simulink subsystem "Day4_5_Scenario_1"  (R2024a)
settings: Solver=VariableStepAuto  StartTime=0.0  StopTime=10.0  RelTol=1e-3
libraries: CarMaker4SL x12, slpidlib x1
settings Model: Creator=junhyung.cha  LastModifiedBy=User

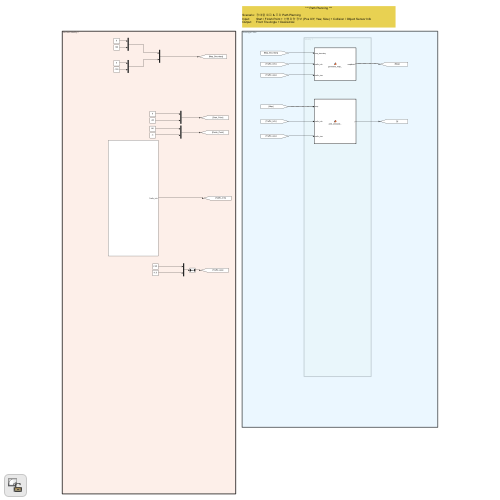
[thumbnail: Simulink's stored preview of the top-level diagram]
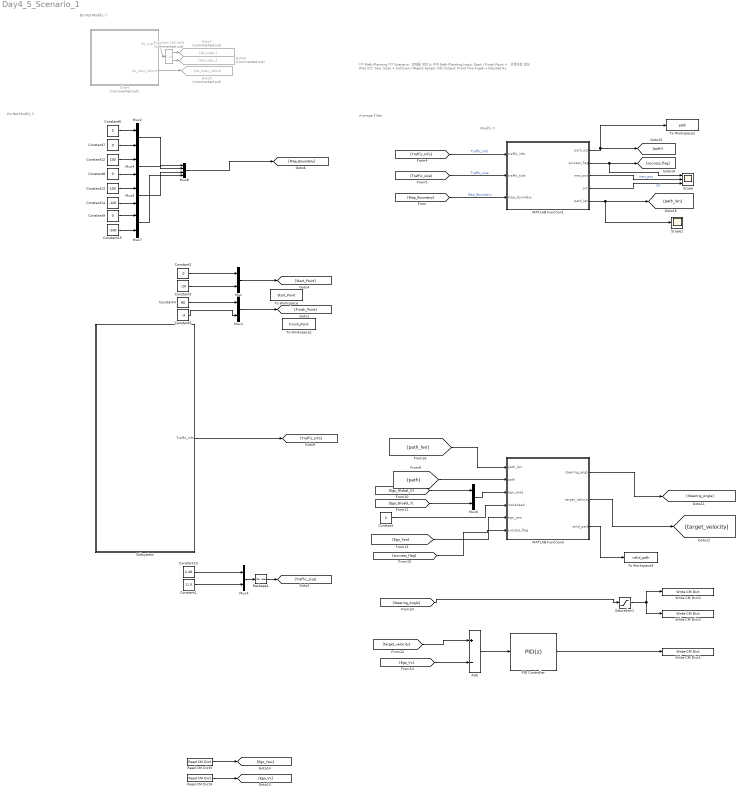
== system Day4_5_Scenario_1 ==
  note: Average Filter
  note: Do Not Modify !!
  note: Modify !!
  note: *** Path Planning ***
      |
      | Scenario: 장애물 회피 & 주차 Path Planning
      | Input: Start / Finish Point + 선행차량 정보 (Pos X/Y, Yaw, Size) + Collision / Object Sensor Info
      | Output: Front Tire Angle + Desired Ax
  note: Do Not Modify !!
  Add : Sum  Inputs=+-
  Chart : Stateflow chart  Commented=on  TreatAsAtomicUnit=on
  Constant : Constant  Value=3
  Constant1 : Constant  Value=11.5
  Constant10 : Constant  Value=2.48
  Constant12 : Constant  Value=100
  Constant13 : Constant  Value=100
  Constant14 : Constant  Value=-100
  Constant15 : Constant  Value=-100
  Constant{2,6..9} (5 alike) : Constant  Value=0
  Constant3 : Constant  Value=-20
  Constant4 : Constant  Value=80
  Constant5 : Constant  Value=-3
  Function-Call Split : FunctionCallSplit  Commented=on  IconShape=distinctive  NumOutputPorts=2  OutputPortLayout=default
  Goto5 : Goto  Commented=on  GotoTag=do_main_10ms
  Goto7 : Goto  Commented=on  GotoTag=do_Logic
  Goto8 : Goto  Commented=on  GotoTag=do_Logic_
  MATLAB Function1 : MATLAB Function  TreatAsAtomicUnit=on
  MATLAB Function3 : MATLAB Function  TreatAsAtomicUnit=on
  Mux{,1..7} (8 alike) : Mux  Inputs=2
  Mux8 : Mux
  PID Controller : slpidlib/PID Controller  Controller=PID  Form=Parallel  TimeDomain=Discrete-time  UseExternalTs=off  SampleTime=-1  IntegratorMethod=Forward Euler  FilterMethod=Forward Euler  ControllerParametersSource=internal  P=3  I=0.01  UseKiTs=off  D=0  UseExternalDerivativeSource=off  N=100  UseFilter=on  TunerSelectOption=Transfer Function Based (PID Tuner App)  InitialConditionSource=internal  InitialConditionForIntegrator=0  InitialConditionForFilter=0  DifferentiatorICPrevScaledInput=0  ExternalReset=none  TrackingMode=off  Kt=1  LimitOutput=off  SatLimitsSource=internal  UpperSaturationLimit=inf  LowerSaturationLimit=-inf  LinearizeAsGain=on  AntiWindupMode=none  Kb=1  LimitIntegrator=off  UpperIntegratorSaturationLimit=inf  LowerIntegratorSaturationLimit=-inf  POutMin=[]  POutMax=[]  IOutMin=[]  IOutMax=[]  DOutMin=[]  DOutMax=[]  NOutMin=[]  NOutMax=[]  SumOutMin=[]  SumOutMax=[]  SaturationOutMin=[]  SaturationOutMax=[]  PParamMin=[]  PParamMax=[]  IParamMin=[]  IParamMax=[]  DParamMin=[]  DParamMax=[]  NParamMin=[]  NParamMax=[]  KbParamMin=[]  KbParamMax=[]  KtParamMin=[]  KtParamMax=[]  KbOutMin=[]  KbOutMax=[]  KtOutMin=[]  KtOutMax=[]  IntegratorOutMin=[]  IntegratorOutMax=[]  FilterOutMin=[]  FilterOutMax=[]  SumI1OutMin=[]  SumI1OutMax=[]  SumI2OutMin=[]  SumI2OutMax=[]  SumI3OutMin=[]  SumI3OutMax=[]  SumI4OutMin=[]  SumI4OutMax=[]  SumDOutMin=[]  SumDOutMax=[]  DifferentiatorOutMin=[]  DifferentiatorOutMax=[]  FilterDiffOutCoefMin=[]  FilterDiffOutCoefMax=[]  ReciprocalOutMin=[]  ReciprocalOutMax=[]  SumDenOutMin=[]  SumDenOutMax=[]  SumNumOutMin=[]  SumNumOutMax=[]  DivideOutMin=[]  DivideOutMax=[]  UdiffTsProdOutMin=[]  UdiffTsProdOutMax=[]  NTsProdOutMin=[]  NTsProdOutMax=[]  UintegralTsProdOutMin=[]  UintegralTsProdOutMax=[]  UngainTsProdOutMin=[]  UngainTsProdOutMax=[]  ClampingZeroOutDataTypeStr=Inherit: Inherit via back propagation  ClampingZeroOutMin=[]  ClampingZeroOutMax=[]  FilterDenConstantOutDataTypeStr=Inherit: Inherit via back propagation  FilterDenConstantOutMin=[]  FilterDenConstantOutMax=[]  PCopyOutDataTypeStr=Inherit: Inherit via back propagation  PCopyOutMin=[]  PCopyOutMax=[]  NCopyOutDataTypeStr=Inherit: Inherit via back propagation  NCopyOutMin=[]  NCopyOutMax=[]  IntegratorContinuousStateAttributes=''  IntegratorStateMustResolveToSignalObject=off  IntegratorRTWStateStorageClass=Auto  FilterContinuousStateAttributes=''  FilterStateMustResolveToSignalObject=off  FilterRTWStateStorageClass=Auto  ParallelPVariant=InternalParameters  IdealPVariant=Disabled  IVariant=InternalParameters  DVariant=InternalParameters  IntegratorVariant=Discrete  SatVariant=Disabled  AWVariant=Passthrough  PCopyVariant=Disabled  TRVariant=Disabled  FdbkBlocksVariant=Forward  IdealPFdbkVariant=Disabled  SatFdbkVariant=Disabled  DerivativeFilterVariant=ForwardEulerFilter  NVariant=InternalParameters  NCopyVariant=Disabled  FilterICVariant=InternalICsFilter  IntegratorICVariant=InternalICs  ExternalResetVariant=Disabled  TRSumVariant=Passthrough  SumFdbkVariant=Disabled  SumVariant=Sum_PID  TsampFilterVariant=InternalTs  TsampNgainVariant=Passthrough  TsampIntegralVariant=Disabled_SignalSpec  ExternalSaturationOutDataTypeStr=Inherit: Same as second input  DerivativeSourceVariant=ErrorSignal
  Read CM Dict3 : CarMaker4SL/Read CM Dict  xname=Car.Fr1.rz  xsync=off  xstime=Inherited
  Read CM Dict4 : CarMaker4SL/Read CM Dict  xname=Car.v  xsync=off  xstime=Inherited
  Reshape1 : Reshape  OutputDimensionality=Row vector (2-D)  OutputDimensions=[2,2]
  Saturation1 : Saturate  UpperLimit=pi/6  LowerLimit=-pi/6
  Scope : Scope  NumInputPorts=3
  Scope1 : Scope
  Subsystem : Subsystem
  To Workspace : ToWorkspace  VariableName=Start_Point  SaveFormat=Structure With Time  SampleTime=-1
  To Workspace1 : ToWorkspace  VariableName=Finish_Point  SaveFormat=Structure With Time  SampleTime=-1
  To Workspace2 : ToWorkspace  VariableName=path  SaveFormat=Structure With Time  SampleTime=-1
  To Workspace3 : ToWorkspace  VariableName=valid_path  SaveFormat=Structure With Time  SampleTime=-1
  Write CM Dict1 : CarMaker4SL/Write CM Dict  xname=AccelCtrl.DesiredAx  xsync=off
  Write CM Dict2 : CarMaker4SL/Write CM Dict  xname=Car.CFL.rz_ext  xsync=off
  Write CM Dict3 : CarMaker4SL/Write CM Dict  xname=Car.CFR.rz_ext  xsync=off
  wires:
  Mux/1 -> [Start_Point]
  Constant2/1 -> Mux/1
  Constant3/1 -> Mux/2
  Constant5/1 -> Mux1/2
  Mux1/1 -> [Finish_Point]
  Constant4/1 -> Mux1/1
  Subsystem/1(Traffic_Info) -> [Traffic_Info]
  Mux3/1 -> Reshape1/1
  Constant10/1 -> Mux3/1
  Constant1/1 -> Mux3/2
  Reshape1/1 -> [Traffic_size]
  Chart/2(do_main_10ms()) -> Goto5/1
  Chart/1(do_Logic()) -> Function-Call Split/1
  Function-Call Split/1 -> Goto7/1
  Function-Call Split/2 -> Goto8/1
  [path] -> MATLAB Function3/2(path)
  Mux6/1 -> MATLAB Function3/3(ego_pose)
  [Ego_Gloabl_Y] -> Mux6/2
  [Ego_Global_X] -> Mux6/1
  Constant/1 -> MATLAB Function3/4(lookahead)
  MATLAB Function3/1(steering_angle) -> [Steering_Angle]
  PID Controller/1 -> Write CM Dict1/1
  [Steering_Angle] -> Saturation1/1
  [Ego_Vx] -> Add/2
  Add/1 -> PID Controller/1
  Saturation1/1 -> Write CM Dict2/1, Write CM Dict3/1
  [target_velocity] -> Add/1
  Constant12/1 -> Mux4/1
  Constant8/1 -> Mux4/2
  Constant6/1 -> Mux2/1
  Constant7/1 -> Mux2/2
  Constant13/1 -> Mux5/1
  Constant14/1 -> Mux5/2
  Constant9/1 -> Mux7/1
  Constant15/1 -> Mux7/2
  Mux2/1 -> Mux8/1
  Mux4/1 -> Mux8/2
  Mux5/1 -> Mux8/3
  Mux7/1 -> Mux8/4
  Mux8/1 -> [Map_Boundary]
  Read CM Dict4/1 -> [Ego_Vx]
  Read CM Dict3/1 -> [Ego_Yaw]
  [Ego_Yaw] -> MATLAB Function3/5(ego_yaw)
  [Traffic_size] -> MATLAB Function1/2(traffic_size)  "Traffic_size"
  [Map_Boundary] -> MATLAB Function1/3(map_boundary)  "Map_Boundary"
  [Traffic_Info] -> MATLAB Function1/1(traffic_info)  "Traffic_Info"
  MATLAB Function1/2(success_flag) -> [success_flag], Scope/1
  MATLAB Function1/1(path_out) -> To Workspace2/1, [path]
  MATLAB Function3/2(target_velocity) -> [target_velocity]
  MATLAB Function1/3(new_pos) -> Scope/2  "new_pos"
  MATLAB Function1/4(cnt) -> Scope/3  "cnt"
  MATLAB Function1/5(path_len) -> [path_len], Scope1/1
  [success_flag] -> MATLAB Function3/6(success_flag)
  [path_len] -> MATLAB Function3/1(path_len)
  MATLAB Function3/3(valid_path) -> To Workspace3/1

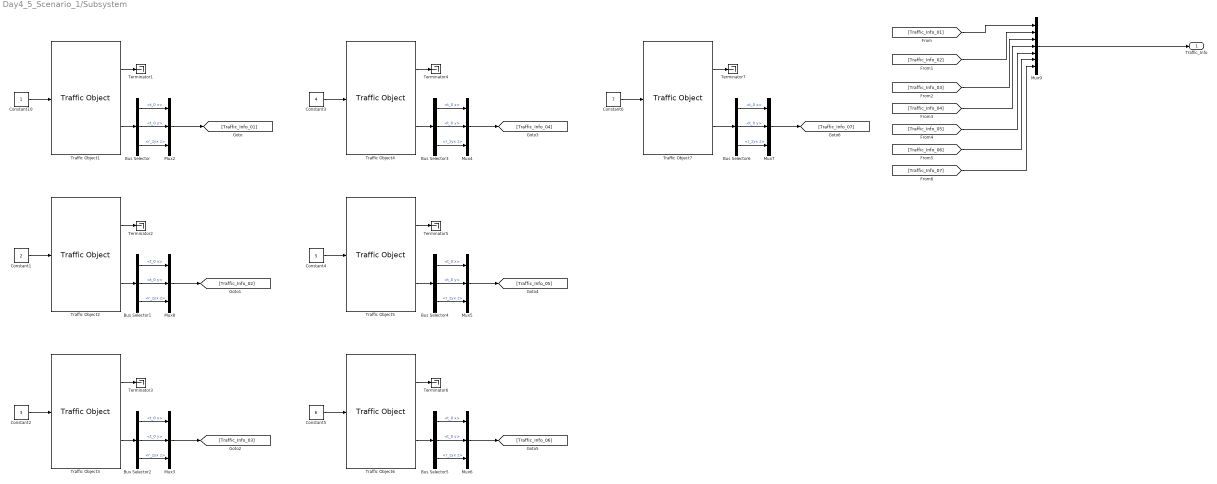
== system Day4_5_Scenario_1/Subsystem ==
  Bus Selector{,1..6} (7 alike) : BusSelector  OutputSignals=t_0 x,t_0 y,r_zyx z
  Constant1 : Constant  Value=2
  Constant10 : Constant
  Constant2 : Constant  Value=3
  Constant3 : Constant  Value=4
  Constant4 : Constant  Value=5
  Constant5 : Constant  Value=6
  Constant6 : Constant  Value=7
  Mux{2..8} (7 alike) : Mux  Inputs=3
  Mux9 : Mux  Inputs=7
  Terminator{1..7} (7 alike) : Terminator
  Traffic Object1 : CarMaker4SL/Traffic Object  xname=T01  ximode=Traffic Id  xstime=Inherited
      settings: SourceProductName=CarMaker4SL
  Traffic Object2 : CarMaker4SL/Traffic Object  xname=T02  ximode=Traffic Id  xstime=Inherited
      settings: SourceProductName=CarMaker4SL
  Traffic Object3 : CarMaker4SL/Traffic Object  xname=T03  ximode=Traffic Id  xstime=Inherited
      settings: SourceProductName=CarMaker4SL
  Traffic Object4 : CarMaker4SL/Traffic Object  xname=T04  ximode=Traffic Id  xstime=Inherited
      settings: SourceProductName=CarMaker4SL
  Traffic Object5 : CarMaker4SL/Traffic Object  xname=T05  ximode=Traffic Id  xstime=Inherited
      settings: SourceProductName=CarMaker4SL
  Traffic Object6 : CarMaker4SL/Traffic Object  xname=T06  ximode=Traffic Id  xstime=Inherited
      settings: SourceProductName=CarMaker4SL
  Traffic Object7 : CarMaker4SL/Traffic Object  xname=T07  ximode=Traffic Id  xstime=Inherited
      settings: SourceProductName=CarMaker4SL
  Traffic_Info : Outport
  wires:
  [Traffic_Info_07] -> Mux9/7
  [Traffic_Info_06] -> Mux9/6
  [Traffic_Info_05] -> Mux9/5
  [Traffic_Info_04] -> Mux9/4
  [Traffic_Info_03] -> Mux9/3
  Mux9/1 -> Traffic_Info/1
  [Traffic_Info_02] -> Mux9/2
  [Traffic_Info_01] -> Mux9/1
  Mux2/1 -> [Traffic_Info_01]
  Traffic Object7/2 -> Bus Selector6/1
  Bus Selector6/3 -> Mux7/3  "<r_zyx z>"
  Bus Selector6/1 -> Mux7/1  "<t_0 x>"
  Mux7/1 -> [Traffic_Info_07]
  Bus Selector6/2 -> Mux7/2  "<t_0 y>"
  Traffic Object6/2 -> Bus Selector5/1
  Bus Selector5/3 -> Mux6/3  "<r_zyx z>"
  Bus Selector5/1 -> Mux6/1  "<t_0 x>"
  Mux6/1 -> [Traffic_Info_06]
  Bus Selector5/2 -> Mux6/2  "<t_0 y>"
  Traffic Object5/2 -> Bus Selector4/1
  Bus Selector4/3 -> Mux5/3  "<r_zyx z>"
  Bus Selector4/1 -> Mux5/1  "<t_0 x>"
  Mux5/1 -> [Traffic_Info_05]
  Bus Selector4/2 -> Mux5/2  "<t_0 y>"
  Traffic Object4/2 -> Bus Selector3/1
  Bus Selector3/3 -> Mux4/3  "<r_zyx z>"
  Bus Selector3/1 -> Mux4/1  "<t_0 x>"
  Mux4/1 -> [Traffic_Info_04]
  Bus Selector3/2 -> Mux4/2  "<t_0 y>"
  Traffic Object3/2 -> Bus Selector2/1
  Bus Selector2/3 -> Mux3/3  "<r_zyx z>"
  Bus Selector2/1 -> Mux3/1  "<t_0 x>"
  Mux3/1 -> [Traffic_Info_03]
  Bus Selector2/2 -> Mux3/2  "<t_0 y>"
  Traffic Object2/2 -> Bus Selector1/1
  Bus Selector1/3 -> Mux8/3  "<r_zyx z>"
  Bus Selector1/1 -> Mux8/1  "<t_0 x>"
  Mux8/1 -> [Traffic_Info_02]
  Bus Selector1/2 -> Mux8/2  "<t_0 y>"
  Bus Selector/3 -> Mux2/3  "<r_zyx z>"
  Bus Selector/2 -> Mux2/2  "<t_0 y>"
  Bus Selector/1 -> Mux2/1  "<t_0 x>"
  Traffic Object1/2 -> Bus Selector/1
  Traffic Object7/1 -> Terminator7/1
  Constant6/1 -> Traffic Object7/1
  Constant5/1 -> Traffic Object6/1
  Traffic Object6/1 -> Terminator6/1
  Traffic Object5/1 -> Terminator5/1
  Constant4/1 -> Traffic Object5/1
  Constant3/1 -> Traffic Object4/1
  Traffic Object4/1 -> Terminator4/1
  Traffic Object3/1 -> Terminator3/1
  Constant2/1 -> Traffic Object3/1
  Constant1/1 -> Traffic Object2/1
  Traffic Object2/1 -> Terminator2/1
  Traffic Object1/1 -> Terminator1/1
  Constant10/1 -> Traffic Object1/1

== matlab function Day4_5_Scenario_1/MATLAB Function3 ==
  settings: updateMethod=DISCRETE  sampleTime=0.1
  data: path_len input; path input; ego_pose input; lookahead input; ego_yaw input; success_flag input; steering_angle output; target_velocity output; valid_path output
function [steering_angle, target_velocity, valid_path] = pure_pursuit_controller(path_len, path, ego_pose, lookahead, ego_yaw, success_flag)
%#codegen

    % 출력 초기화
    steering_angle = 0.0;
    target_velocity = 0.0;
    valid_path = zeros(100, 2);  % 고정 크기

    % 경로가 유효하지 않으면 → 무조건 0 유지
    if ~success_flag || path_len < 1
        % 모든 출력 명시적으로 0 유지
        steering_angle = 0.0;
        target_velocity = 0.0;
        valid_path(:,:) = 0.0;
        return;
    end

    % path_len만큼만 유효 경로 복사
    valid_path(1:path_len, :) = path(1:path_len, :);

    % 자차 위치 및 자세
    x = ego_pose(1);
    y = ego_pose(2);
    yaw = ego_yaw;

    % 로컬 좌표계로 변환
    path_local = zeros(path_len, 2);
    for i = 1:path_len
        dx = valid_path(i,1) - x;
        dy = valid_path(i,2) - y;
        path_local(i,1) = cos(-yaw)*dx - sin(-yaw)*dy;
        path_local(i,2) = sin(-yaw)*dx + cos(-yaw)*dy;
    end

    % 기본 타겟은 마지막 점
    target = path_local(path_len, :);
    for i = 1:path_len
        if hypot(path_local(i,1), path_local(i,2)) > lookahead
            target = path_local(i,:);
            break;
        end
    end

    % 조향각 및 속도 계산
    L = 2.5;
    x_r = target(1);
    y_r = target(2);

    if x_r > 0
        steering_angle = atan2(2 * L * y_r, lookahead^2);
        target_velocity = 30 / 3.6;  % 30km/h
    else
        % 전방 타겟이 없을 경우 → 정지 유지
        steering_angle = 0.0;
        target_velocity = 0.0;
    end
end
% 
% function [steering_angle, target_velocity] = pure_pursuit_controller(path_len, path, ego_pose, lookahead, ego_yaw, success_flag)
% #codegen
% 
%     기본 출력값 초기화 (Simulink 필수)
%     steering_angle = 0.0;
%     target_velocity = 0.0;
% 
%     자차 위치
%     x = ego_pose(1);
%     y = ego_pose(2);
%     yaw = ego_yaw;
% 
%     유효 경로 길이 확인
%     if path_len < 1
%         return;
%     end
% 
%     유효한 경로만 추출
%     valid_path = path(1:path_len, :);
% 
%     fallback: 마지막 경로점으로 초기화
%     target = valid_path(end, :);
% 
%     lookahead 거리 이상 앞에 있는 점 찾기
%     for i = 1:path_len
%         dx = valid_path(i,1) - x;
%         dy = valid_path(i,2) - y;
%         dist = hypot(dx, dy);
%         x_r = cos(-yaw)*dx - sin(-yaw)*dy;
% 
%         if dist > lookahead && x_r > 0
%             target = valid_path(i,:);
%             break;
%         end
%     end
% 
%     자차 기준 좌표로 변환
%     dx = target(1) - x;
%     dy = target(2) - y;
%     x_r = cos(-yaw)*dx - sin(-yaw)*dy;
%     y_r = sin(-yaw)*dx + cos(-yaw)*dy;
% 
%     조향각 계산 (wheelbase = 2.5 assumed)
%     L = 2.5;
%     if success_flag && x_r ~= 0
%         steering_angle = atan2(2 * L * y_r, lookahead^2);
%         target_velocity = 30 / 3.6;
%     end
% end

== stateflow chart Day4_5_Scenario_1/Chart ==
  (default) -> (junction 1)
  (junction 1) -> (junction 3) [order 1] : [i<99]
      | {i = i + 1;}
  (junction 1) -> (junction 7) [order 2] : {i=0;}
  (junction 3) -> (junction 5)
  (junction 5) -> (junction 7)
  (junction 7) -> (junction 10)
  (junction 10) -> (junction 12) [order 1] : [rem(i,50) == 0]
      | {do_Logic;}
  (junction 10) -> (junction 18) [order 2]
  (junction 12) -> (junction 16)
  (junction 16) -> (junction 18)
  (junction 18) -> (junction 27)
  (junction 27) -> (junction 29) [order 1] : [rem(i,10) == 0]
      | {do_main_10ms}
  (junction 29) -> (junction 33)
  (junction 27) -> (junction 21) [order 2]
  (junction 33) -> (junction 21)
  (junction 21) -> (junction 41)
  data: i local =0
  events: do_Logic output FUNCTION_CALL_EVENT; do_main_10ms output FUNCTION_CALL_EVENT

== matlab function Day4_5_Scenario_1/MATLAB Function1 ==
  settings: updateMethod=DISCRETE  sampleTime=0.1
  data: traffic_info input; traffic_size input; path_out output; success_flag output; new_pos output; cnt output; map_boundary input; path_len output
% 최종 안정화된 RRT* + Simulink 캐시 버전
function [path_out, success_flag, new_pos, cnt, path_len] = rrt_star_simulink(traffic_info, traffic_size, map_boundary)
%#codegen

%% Persistent 캐시로 path 재탐색 방지
persistent path_cached path_len_cached success_cached

% 캐시 초기화 (Simulink 요구사항)
if isempty(path_cached)
    path_cached = zeros(100, 2); % MAX_PATH_LEN
    path_len_cached = 0;
    success_cached = false;
end

% 출력 초기화
path_out = path_cached;
path_len = path_len_cached;
success_flag = success_cached;
new_pos = zeros(1,2);
cnt = 0;

% 경로가 이미 성공했으면 캐시된 값 반환
if success_cached
    return;
end

%% 파라미터 설정
MAX_NODES = 1000;
MAX_PATH_LEN = 100;
goal_range = 2.0;
goal_sample_rate = 0.05;
eta = 3.0;

start = [0.0, -20.0];
goal  = [80.0, -3.0];
vehicle_size = traffic_size;

%% 맵 범위 설정
x_vals = map_boundary(1:2:end);
y_vals = map_boundary(2:2:end);
x_min = min(x_vals); x_max = max(x_vals);
y_min = min(y_vals); y_max = max(y_vals);

%% 장애물 구성
num_obj = length(traffic_info)/3;
data = reshape(traffic_info, [3, num_obj])';
data(1:4,1:2) = data(1:4,1:2) + [-1.24, +5.75];
data(5:7,1:2) = data(5:7,1:2) + [4.27, 0];
obstacles = [data(:,1:2), repmat(traffic_size, num_obj, 1), data(:,3)];

%% 노드 구조체 초기화
empty_node = struct('pos', zeros(1,2), 'cost', 0, 'parent', int32(0));
nodes = repmat(empty_node, MAX_NODES, 1);
nodes(1).pos = start;
nodes(1).cost = 0;
nodes(1).parent = int32(0);
node_count = int32(1);
goal_node = int32(0);

%% RRT* 탐색 루프
for iter = 1:500
    % 샘플링
    if rand < goal_sample_rate
        sample = goal;
    else
        sample = [x_min + rand*(x_max - x_min), y_min + rand*(y_max - y_min)];
    end

    % 최근접 노드 탐색
    nearest_idx = int32(1);
    min_dist = norm(nodes(1).pos - sample);
    for i = 2:node_count
        d = norm(nodes(i).pos - sample);
        if d < min_dist
            min_dist = d;
            nearest_idx = int32(i);
        end
    end

    % 방향 설정
    direction = sample - nodes(nearest_idx).pos;
    dist = norm(direction);
    if dist > eta
        direction = direction / dist * eta;
    end
    new_pos = nodes(nearest_idx).pos + direction;

    % 충돌 체크
    if check_collision(nodes(nearest_idx).pos, new_pos, vehicle_size, obstacles)
        cnt = cnt + 1;
        continue;
    end

    % 새 노드 추가
    node_count = node_count + 1;
    if node_count > MAX_NODES
        break;
    end
    nodes(node_count).pos = new_pos;
    nodes(node_count).cost = nodes(nearest_idx).cost + dist;
    nodes(node_count).parent = nearest_idx;

    % 종료 조건
    if norm(new_pos - goal) < goal_range
        goal_node = node_count;
        break;
    end
end

%% 경로 복원
if goal_node > 0
    idx = goal_node;
    i = 0;
    temp_path = zeros(MAX_PATH_LEN, 2);
    while idx > 0 && i < MAX_PATH_LEN
        i = i + 1;
        temp_path(i,:) = nodes(idx).pos;
        idx = nodes(idx).parent;
    end
    path_out = zeros(MAX_PATH_LEN, 2);
    path_out(1:i,:) = flipud(temp_path(1:i,:));
    path_len = i;
    success_flag = true;

    % ✅ 캐시에 저장
    path_cached = path_out;
    path_len_cached = path_len;
    success_cached = true;
end
end

%% 충돌 체크 함수
function collision = check_collision(p1, p2, vehicle_size, obs_list)
    collision = false;
    steps = 10;
    for t = linspace(0,1,steps)
        pt = (1-t)*p1 + t*p2;
        yaw = atan2(p2(2)-p1(2), p2(1)-p1(1));
        veh = get_bbox(pt, yaw, vehicle_size);
        for i = 1:size(obs_list,1)
            obs = get_bbox(obs_list(i,1:2), obs_list(i,5), obs_list(i,3:4));
            if box_overlap(veh, obs)
                collision = true;
                return;
            end
        end
    end
end

%% 사각형 구성 함수
function box = get_bbox(center, yaw, size)
    w = size(1); h = size(2);
    dx = [ w/2, -w/2, -w/2,  w/2];
    dy = [ h/2,  h/2, -h/2, -h/2];
    R = [cos(yaw), -sin(yaw); sin(yaw), cos(yaw)];
    temp = R * [dx; dy];
    box = temp + center';
end

%% SAT (Separating Axis Theorem)
function overlap = box_overlap(b1, b2)
    overlap = true;
    axes = get_axes(b1, b2);
    for i = 1:size(axes,2)
        proj1 = axes(:,i)' * b1;
        proj2 = axes(:,i)' * b2;
        if max(proj1) < min(proj2) || max(proj2) < min(proj1)
            overlap = false;
            return;
        end
    end
end

function axes = get_axes(b1, b2)
    edges = [b1(:,2)-b1(:,1), b1(:,3)-b1(:,2)];
    normals = [-edges(2,:); edges(1,:)];
    axes = normals ./ vecnorm(normals);
end
